simulink model "door_lock_system"  (R2018a)
settings: Solver=FixedStepDiscrete  StartTime=0.0  StopTime=10.0  FixedStep=1  RelTol=1e-3
undefined symbols (not defined in the file or in its folder): carlight, doorlockstatus, taillight
libraries: simulink x7
settings Model: Creator=sagar  LastModifiedBy=sagar
settings ConfigComp: CovEnable=on  CovScope=ReferencedModels  RecordCoverage=on

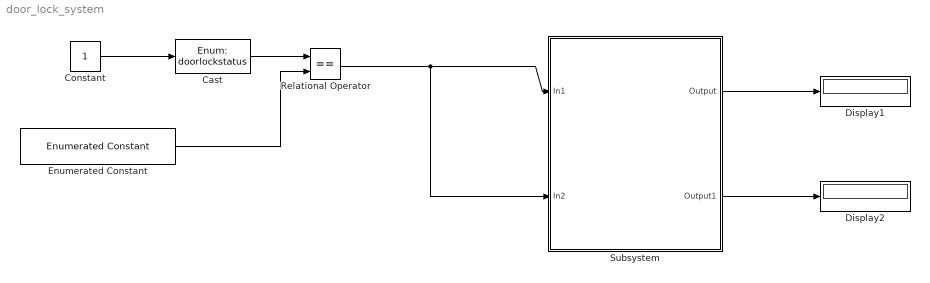
== system door_lock_system ==
  Cast : DataTypeConversion  OutDataTypeStr=Enum: doorlockstatus
  Constant : Constant  OutDataTypeStr=uint8
  Display1 : Display
  Display2 : Display
  Enumerated Constant : simulink/Sources/Enumerated Constant  OutDataTypeStr=Enum: doorlockstatus  Value=doorlockstatus.door_lock_close  SampleTime=inf
      settings: SourceProductName=Simulink
  Relational Operator : RelationalOperator  Operator===  OutDataTypeStr=boolean  RndMeth=Simplest
  Subsystem : Subsystem
  wires:
  Enumerated Constant/1 -> Relational Operator/2
  Cast/1 -> Relational Operator/1
  Constant/1 -> Cast/1
  Relational Operator/1 -> Subsystem/2(In2), Subsystem/1(In1)
  Subsystem/1(Output) -> Display1/1
  Subsystem/2(Output1) -> Display2/1

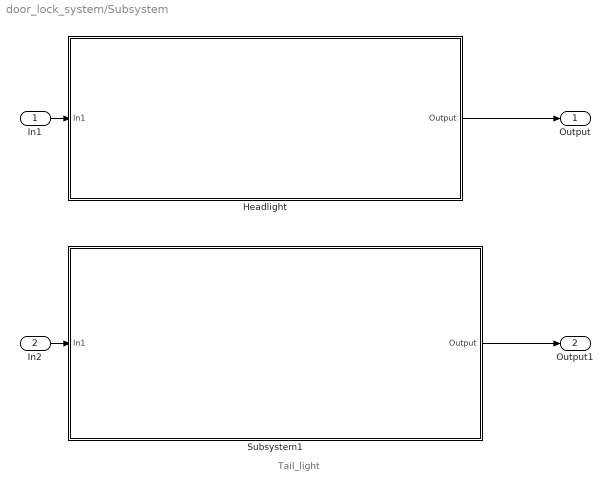
== system door_lock_system/Subsystem ==
  note: Tail_light
  In1 : Inport
  In2 : Inport  Port=2
  Headlight : Subsystem
  Subsystem1 : Subsystem
  Output : Outport
  Output1 : Outport  Port=2
  wires:
  In1/1 -> Headlight/1(In1)
  In2/1 -> Subsystem1/1(In1)
  Headlight/1(Output) -> Output/1
  Subsystem1/1(Output) -> Output1/1

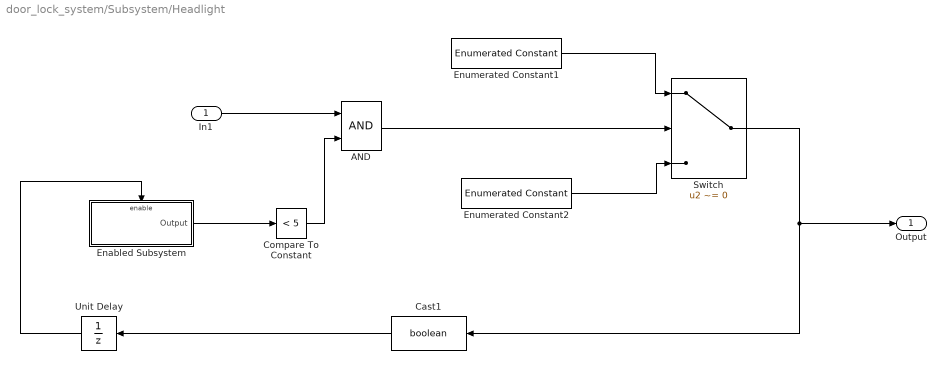
== system door_lock_system/Subsystem/Headlight ==
  In1 : Inport
  AND : Logic  AllPortsSameDT=off  OutDataTypeStr=boolean
  Cast1 : DataTypeConversion  OutDataTypeStr=boolean
  Compare To Constant : simulink/Logic and Bit Operations/Compare To Constant  relop=<  const=5  OutDataTypeStr=boolean
  Enabled Subsystem : Subsystem  TreatAsAtomicUnit=on
  Enumerated Constant1 : simulink/Sources/Enumerated Constant  OutDataTypeStr=Enum: carlight  Value=carlight.Head_light_on  SampleTime=inf
      settings: SourceProductName=Simulink
  Enumerated Constant2 : simulink/Sources/Enumerated Constant  OutDataTypeStr=Enum: carlight  Value=carlight.Head_light_off  SampleTime=inf
      settings: SourceProductName=Simulink
  Switch : Switch  Criteria=u2 ~= 0
  Unit Delay : UnitDelay  SampleTime=-1
  Output : Outport
  wires:
  Switch/1 -> Output/1, Cast1/1
  In1/1 -> AND/1
  Enumerated Constant2/1 -> Switch/3
  Enabled Subsystem/1(Output) -> Compare To Constant/1
  Unit Delay/1 -> Enabled Subsystem/Enable
  AND/1 -> Switch/2
  Cast1/1 -> Unit Delay/1
  Enumerated Constant1/1 -> Switch/1
  Compare To Constant/1 -> AND/2

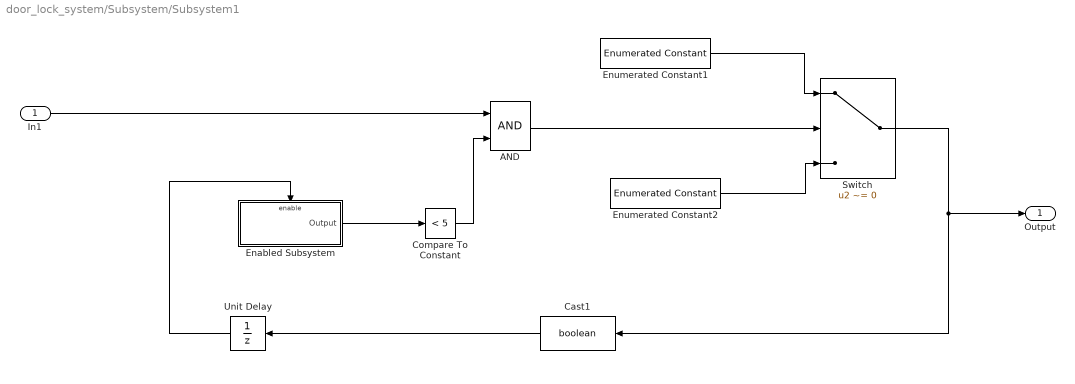
== system door_lock_system/Subsystem/Subsystem1 ==
  In1 : Inport
  AND : Logic  AllPortsSameDT=off  OutDataTypeStr=boolean
  Cast1 : DataTypeConversion  OutDataTypeStr=boolean
  Compare To Constant : simulink/Logic and Bit Operations/Compare To Constant  relop=<  const=5  OutDataTypeStr=boolean
  Enabled Subsystem : Subsystem  TreatAsAtomicUnit=on
  Enumerated Constant1 : simulink/Sources/Enumerated Constant  OutDataTypeStr=Enum: taillight  Value=taillight.tail_light_on  SampleTime=inf
      settings: SourceProductName=Simulink
  Enumerated Constant2 : simulink/Sources/Enumerated Constant  OutDataTypeStr=Enum: taillight  Value=taillight.tail_light_off  SampleTime=inf
      settings: SourceProductName=Simulink
  Switch : Switch  Criteria=u2 ~= 0
  Unit Delay : UnitDelay  SampleTime=-1
  Output : Outport
  wires:
  Enabled Subsystem/1(Output) -> Compare To Constant/1
  AND/1 -> Switch/2
  Unit Delay/1 -> Enabled Subsystem/Enable
  In1/1 -> AND/1
  Compare To Constant/1 -> AND/2
  Enumerated Constant1/1 -> Switch/1
  Enumerated Constant2/1 -> Switch/3
  Cast1/1 -> Unit Delay/1
  Switch/1 -> Output/1, Cast1/1

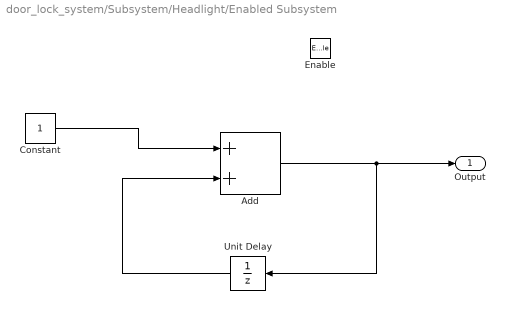
== system door_lock_system/Subsystem/Headlight/Enabled Subsystem ==
  Enable : EnablePort
  Add : Sum
  Constant : Constant
  Unit Delay : UnitDelay  SampleTime=-1
  Output : Outport
  wires:
  Add/1 -> Output/1, Unit Delay/1
  Constant/1 -> Add/1
  Unit Delay/1 -> Add/2

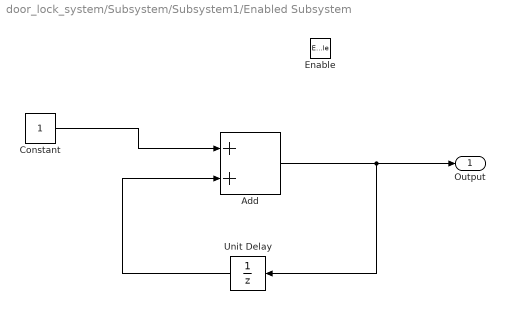
== system door_lock_system/Subsystem/Subsystem1/Enabled Subsystem ==
  Enable : EnablePort
  Add : Sum
  Constant : Constant
  Unit Delay : UnitDelay  SampleTime=-1
  Output : Outport
  wires:
  Add/1 -> Output/1, Unit Delay/1
  Constant/1 -> Add/1
  Unit Delay/1 -> Add/2
